simulink model "Stop_and_Wait"  (R2023b)
settings: Solver=VariableStepAuto  StartTime=0.0  StopTime=10.0  RelTol=1e-3
libraries: dspnetwork x2
settings Model: Creator=Amin  LastModifiedBy=Amin

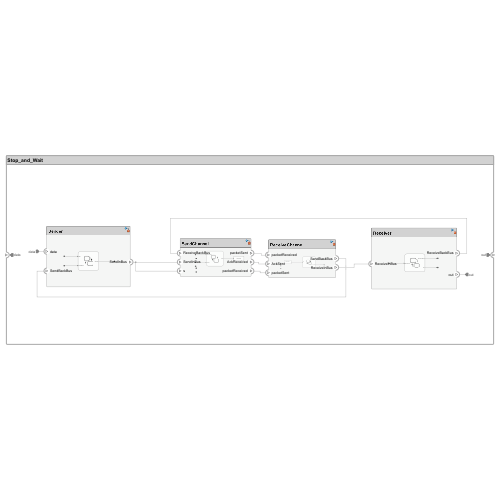
[thumbnail: Simulink's stored preview of the top-level diagram]
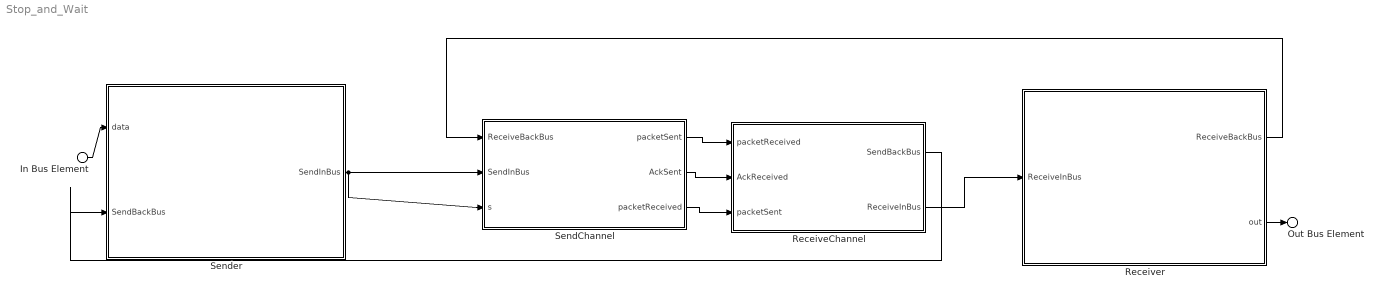
== system Stop_and_Wait ==
  In Bus Element : Inport  PortName=data
  ReceiveChannel : Subsystem
      settings: PortSchema="{\"entries\":[{\"content\":{\"headerSize\":26,\"margin\":15,\"minimumSpacing\":25,\"sides\":[{\"content\":{\"connectorIds\":[\"In1\",\"In2\",\"In3\"]},\"type\":\"ConnectorPlacement.EquallySpacedRectSide\",\"uuid\":\"304fcf97-283e-4d15-a872-e521c327b52d\"},{\"content\":{\"connectorIds\":[\"Out1\",\"Out2\"],\"side\":\"RIGHT\"},\"type\":\"ConnectorPlacement.EquallySpacedRectSide\",\"uuid\":\"74835837-8d51-451b-8cd4-fc2a54f63838\"},{\"content\":{\"side\":\"TOP\"},\"type\":\"ConnectorPlacement.EquallySpacedRectSide\",\"uuid\":\"e554d6ec-8da4-46f0-8d11-e5ada8ab82dd\"}]},\"type\":\"ConnectorPlacement.EquallySpacedConnector\",\"uuid\":\"b2373ef1-a199-4f6f-9fb7-9087cc4a378d\"}],\"packageUris\":[\"http://schema.mathworks.com/mf0/Connector/R2020b\"],\"version\":\"1.0\"}"
  Receiver : Subsystem
      settings: PortSchema="{\"entries\":[{\"content\":{\"headerSize\":26,\"margin\":15,\"minimumSpacing\":25,\"sides\":[{\"content\":{\"connectorIds\":[\"In1\"]},\"type\":\"ConnectorPlacement.EquallySpacedRectSide\",\"uuid\":\"469fc166-a806-4e78-979e-db8d95df498e\"},{\"content\":{\"connectorIds\":[\"Out1\",\"Out2\"],\"side\":\"RIGHT\"},\"type\":\"ConnectorPlacement.EquallySpacedRectSide\",\"uuid\":\"17031e56-185c-4bae-8c71-286a1fdd36a8\"},{\"content\":{\"side\":\"TOP\"},\"type\":\"ConnectorPlacement.EquallySpacedRectSide\",\"uuid\":\"a4955088-a9ee-4ca0-ba88-780b92c6cbcb\"}]},\"type\":\"ConnectorPlacement.EquallySpacedConnector\",\"uuid\":\"c8c58f11-4281-4cb3-8e8d-2e4eb6673e4e\"}],\"packageUris\":[\"http://schema.mathworks.com/mf0/Connector/R2020b\"],\"version\":\"1.0\"}"
  SendChannel : Subsystem
      settings: PortSchema="{\"entries\":[{\"content\":{\"headerSize\":26,\"margin\":15,\"minimumSpacing\":25,\"sides\":[{\"content\":{\"connectorIds\":[\"In1\",\"In2\",\"In3\"]},\"type\":\"ConnectorPlacement.EquallySpacedRectSide\",\"uuid\":\"469fc166-a806-4e78-979e-db8d95df498e\"},{\"content\":{\"connectorIds\":[\"Out1\",\"Out2\",\"Out3\"],\"side\":\"RIGHT\"},\"type\":\"ConnectorPlacement.EquallySpacedRectSide\",\"uuid\":\"17031e56-185c-4bae-8c71-286a1fdd36a8\"},{\"content\":{\"side\":\"TOP\"},\"type\":\"ConnectorPlacement.EquallySpacedRectSide\",\"uuid\":\"a4955088-a9ee-4ca0-ba88-780b92c6cbcb\"}]},\"type\":\"ConnectorPlacement.EquallySpacedConnector\",\"uuid\":\"c8c58f11-4281-4cb3-8e8d-2e4eb6673e4e\"}],\"packageUris\":[\"http://schema.mathworks.com/mf0/Connector/R2020b\"],\"version\":\"1.0\"}"
  Sender : Subsystem
      settings: PortSchema="{\"entries\":[{\"content\":{\"headerSize\":26,\"margin\":15,\"minimumSpacing\":25,\"sides\":[{\"content\":{\"connectorIds\":[\"In1\",\"In2\"]},\"type\":\"ConnectorPlacement.EquallySpacedRectSide\",\"uuid\":\"a0fda4bb-c687-4862-af45-71af529babf1\"},{\"content\":{\"connectorIds\":[\"Out1\"],\"side\":\"RIGHT\"},\"type\":\"ConnectorPlacement.EquallySpacedRectSide\",\"uuid\":\"bf3aa4ba-14b7-45bd-8425-10615cda76cd\"},{\"content\":{\"side\":\"TOP\"},\"type\":\"ConnectorPlacement.EquallySpacedRectSide\",\"uuid\":\"cc07c9b4-11d7-4695-b3d1-072a460ecc5c\"}]},\"type\":\"ConnectorPlacement.EquallySpacedConnector\",\"uuid\":\"6dd78809-7abd-43f1-9c2f-f4549f98139f\"}],\"packageUris\":[\"http://schema.mathworks.com/mf0/Connector/R2020b\"],\"version\":\"1.0\"}"
  Out Bus Element : Outport  PortName=out
  wires:
  Sender/1(SendInBus) -> SendChannel/3(s), SendChannel/2(SendInBus)
  Receiver/1(ReceiveBackBus) -> SendChannel/1(ReceiveBackBus)
  Receiver/2(out) -> Out Bus Element/1
  In Bus Element/1 -> Sender/1(data)
  ReceiveChannel/2(ReceiveInBus) -> Receiver/1(ReceiveInBus)
  ReceiveChannel/1(SendBackBus) -> Sender/2(SendBackBus)
  SendChannel/1(packetSent) -> ReceiveChannel/1(packetReceived)
  SendChannel/2(AckSent) -> ReceiveChannel/2(AckReceived)
  SendChannel/3(packetReceived) -> ReceiveChannel/3(packetSent)

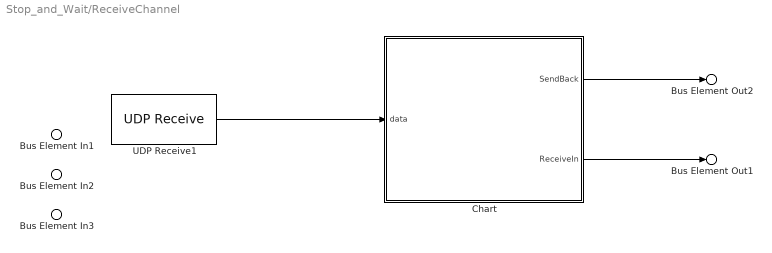
== system Stop_and_Wait/ReceiveChannel ==
  Bus Element In1 : Inport  PortName=packetReceived
  Bus Element In2 : Inport  Port=2  PortName=AckReceived
  Bus Element In3 : Inport  Port=3  PortName=packetSent
  Chart : Stateflow chart  TreatAsAtomicUnit=on
  UDP Receive1 : dspnetwork/UDP Receive  localURL='0.0.0.0'  localPort=25000  remoteURL='0.0.0.0'  remotePort=-1  recvBufferSize=8192  dims=255  signalDatatype=uint8  isComplex=off  isVarSize=on  showBlockingTime=off  blockingTime=0  sampletime=1  blockPlatform=[]
      settings: LibrarySourceBlock=dspsrcs4/UDP Receive
  Bus Element Out2 : Outport  PortName=SendBackBus
  Bus Element Out1 : Outport  Port=2  PortName=ReceiveInBus
  wires:
  Chart/1(SendBack) -> Bus Element Out2/1
  Chart/2(ReceiveIn) -> Bus Element Out1/1
  UDP Receive1/1 -> Chart/1(data)

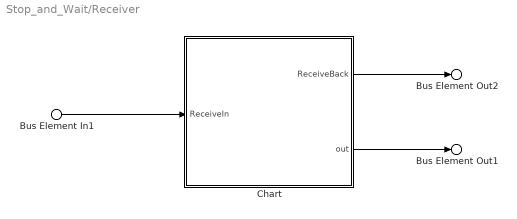
== system Stop_and_Wait/Receiver ==
  Bus Element In1 : Inport  PortName=ReceiveInBus
  Chart : Stateflow chart  TreatAsAtomicUnit=on
  Bus Element Out2 : Outport  PortName=ReceiveBackBus
  Bus Element Out1 : Outport  Port=2  PortName=out
  wires:
  Bus Element In1/1 -> Chart/1(ReceiveIn)
  Chart/1(ReceiveBack) -> Bus Element Out2/1
  Chart/2(out) -> Bus Element Out1/1

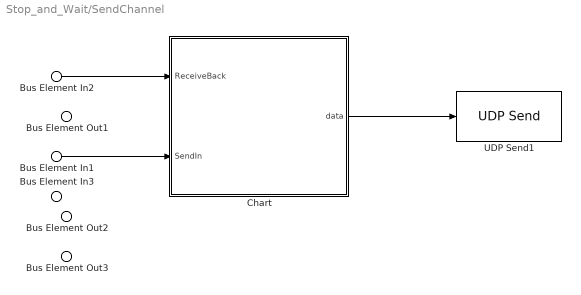
== system Stop_and_Wait/SendChannel ==
  Bus Element In2 : Inport  PortName=ReceiveBackBus
  Bus Element In1 : Inport  Port=2  PortName=SendInBus
  Bus Element In3 : Inport  Port=3  PortName=s
  Chart : Stateflow chart  TreatAsAtomicUnit=on
  UDP Send1 : dspnetwork/UDP Send  remoteURL='127.0.0.1'  remotePort=25000  localURL='0.0.0.0'  localPortSource=Automatically determine  localPort=-1  sendBufferSize=8192  sampletime=-1  blockPlatform=[]  separateLengthPort=0
      settings: LibrarySourceBlock=dspsnks4/UDP Send
  Bus Element Out1 : Outport  PortName=packetSent
  Bus Element Out2 : Outport  Port=2  PortName=AckSent
  Bus Element Out3 : Outport  Port=3  PortName=packetReceived
  wires:
  Bus Element In1/1 -> Chart/2(SendIn)
  Bus Element In2/1 -> Chart/1(ReceiveBack)
  Chart/1(data) -> UDP Send1/1

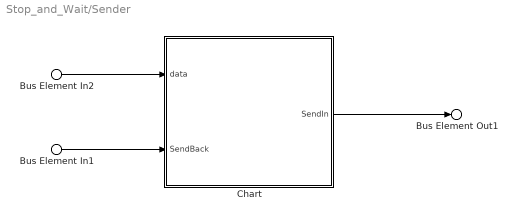
== system Stop_and_Wait/Sender ==
  Bus Element In2 : Inport  PortName=data
  Bus Element In1 : Inport  Port=2  PortName=SendBackBus
  Chart : Stateflow chart  TreatAsAtomicUnit=on
  Bus Element Out1 : Outport  PortName=SendInBus
  wires:
  Chart/1(SendIn) -> Bus Element Out1/1
  Bus Element In2/1 -> Chart/1(data)
  Bus Element In1/1 -> Chart/2(SendBack)

== stateflow chart Stop_and_Wait/Receiver/Chart ==
  data: ReceiveIn input; ReceiveBack output; out output

== stateflow chart Stop_and_Wait/ReceiveChannel/Chart ==
  data: data input size=255; SendBack output; ReceiveIn output

== stateflow chart Stop_and_Wait/Sender/Chart ==
  data: SendIn output; data input; SendBack input

== stateflow chart Stop_and_Wait/SendChannel/Chart ==
  data: ReceiveBack input; SendIn input; data output
